simulink model "PropellerDynamics"  (R2024b)
settings: configuration reference "VTOLConfiguration" (kept outside this file)
undefined symbols (not defined in the file): minPWM, uavParam
libraries: sharedutil x2
settings Model: DataDictionary=VTOLDynamicsData.sldd  Creator=The MathWorks, Inc.  LastModifiedBy=jjha
settings ConfigSetRef: SourceName=VTOLConfiguration

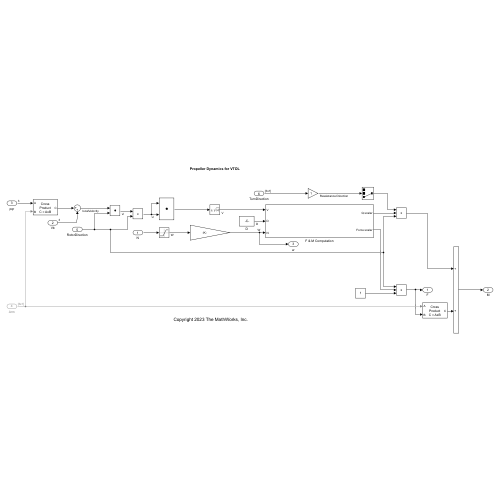
[thumbnail: Simulink's stored preview of the top-level diagram]
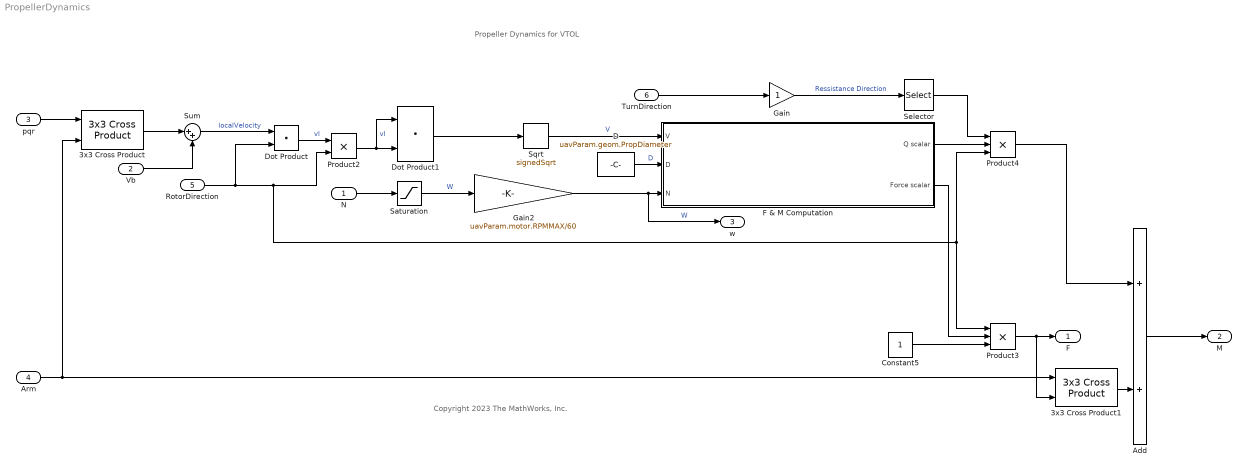
== system PropellerDynamics ==
  note: Propeller Dynamics for VTOL
  note: Copyright 2023 The MathWorks, Inc.
  N : Inport  OutDataTypeStr=double  PortDimensions=1
  Vb : Inport  Port=2  PortDimensions=3
  pqr : Inport  Port=3  PortDimensions=3
  Arm : Inport  Port=4  PortDimensions=[3 1]
  RotorDirection : Inport  Port=5
  TurnDirection : Inport  Port=6  PortDimensions=[3 1]
  3x3 Cross Product : sharedutil/3x3 Cross Product  aMode=aMode
  3x3 Cross Product1 : sharedutil/3x3 Cross Product  aMode=aMode
  Add : Sum
  Constant5 : Constant
  D : Constant  Value=uavParam.geom.PropDiameter
  Dot Product : DotProduct  OutDataTypeStr=Inherit: Inherit via internal rule
  Dot Product1 : DotProduct  OutDataTypeStr=Inherit: Inherit via internal rule
  F & M Computation : Subsystem
  Gain : Gain
  Gain2 : Gain  Gain=uavParam.motor.RPMMAX/60
  Product2 : Product
  Product3 : Product  Inputs=3
  Product4 : Product  Inputs=3
  Saturation : Saturate  UpperLimit=1  LowerLimit=minPWM
  Selector : Selector  InputPortWidth=3  IndexOptions=Index vector (dialog)  Indices=3  OutputSizes=1
  Sqrt : Sqrt  Operator=signedSqrt
  Sum : Sum  Inputs=|++
  F : Outport
  M : Outport  Port=2
  w : Outport  Port=3
  wires:
  3x3 Cross Product1/1 -> Add/2
  Sum/1 -> Dot Product/1  "localVelocity"
  N/1 -> Saturation/1
  pqr/1 -> 3x3 Cross Product/1
  Gain/1 -> Selector/1  "Ressistance Direction"
  Arm/1 -> 3x3 Cross Product/2, 3x3 Cross Product1/1
  Dot Product/1 -> Product2/1  "vl"
  3x3 Cross Product/1 -> Sum/1
  F & M Computation/2(Force scalar) -> Product3/2
  Vb/1 -> Sum/2
  RotorDirection/1 -> Product3/1, Product4/3, Product2/2, Dot Product/2
  Product2/1 -> Dot Product1/2, Dot Product1/1  "vl"
  Saturation/1 -> Gain2/1  "W"
  TurnDirection/1 -> Gain/1
  Dot Product1/1 -> Sqrt/1
  Sqrt/1 -> F & M Computation/1(V)  "V"
  D/1 -> F & M Computation/2(D)  "D"
  F & M Computation/1(Q scalar) -> Product4/2
  Selector/1 -> Product4/1
  Product3/1 -> 3x3 Cross Product1/2, F/1
  Constant5/1 -> Product3/3
  Product4/1 -> Add/1
  Add/1 -> M/1
  Gain2/1 -> w/1, F & M Computation/3(N)  "W"

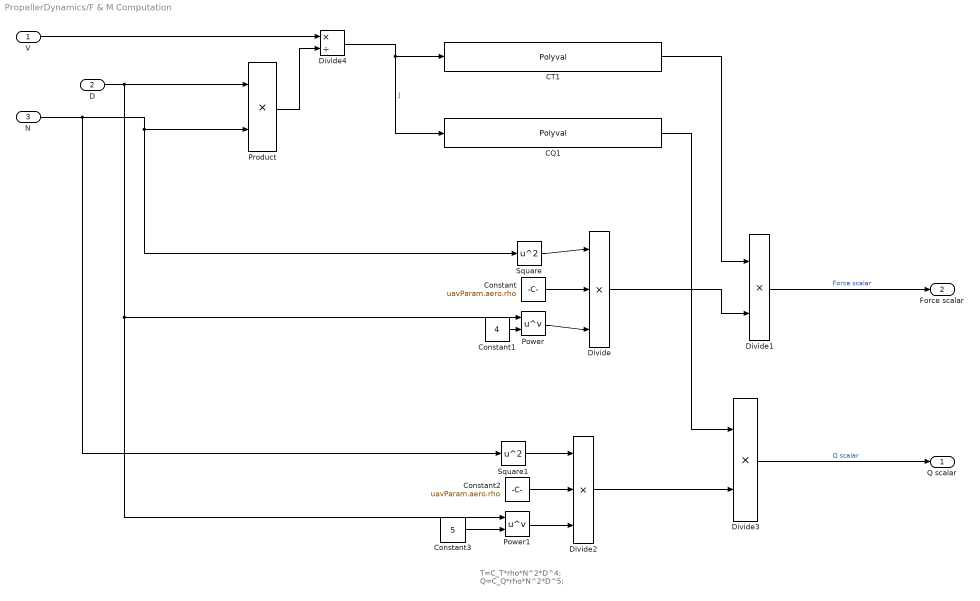
== system PropellerDynamics/F & M Computation ==
  note: T=C_T*rho*N^2*D^4;
      | Q=C_Q*rho*N^2*D^5;
  V : Inport
  D : Inport  Port=2
  N : Inport  Port=3
  CQ1 : Polyval  Coefs=[0.04280,-0.05046,0.005711,-0.003293, 0.007048]
  CT1 : Polyval  Coefs=[0.03338, -0.1265,-0.1210,0.1142]
  Constant : Constant  Value=uavParam.aero.rho
  Constant1 : Constant  Value=4
  Constant2 : Constant  Value=uavParam.aero.rho
  Constant3 : Constant  Value=5
  Divide : Product  Inputs=***
  Divide1 : Product  Inputs=**
  Divide2 : Product  Inputs=***
  Divide3 : Product  Inputs=**
  Divide4 : Product  Inputs=*/
  Power : Math  Operator=pow
  Power1 : Math  Operator=pow
  Product : Product
  Square : Math  Operator=square
  Square1 : Math  Operator=square
  Q scalar : Outport
  Force scalar : Outport  Port=2
  wires:
  Divide4/1 -> CQ1/1, CT1/1  "J"
  Product/1 -> Divide4/2
  CT1/1 -> Divide1/1
  Divide2/1 -> Divide3/2
  CQ1/1 -> Divide3/1
  Divide3/1 -> Q scalar/1  "Q scalar"
  Divide/1 -> Divide1/2
  Divide1/1 -> Force scalar/1  "Force scalar"
  V/1 -> Divide4/1
  Power/1 -> Divide/3
  Constant/1 -> Divide/2
  Constant3/1 -> Power1/2
  Square/1 -> Divide/1
  Power1/1 -> Divide2/3
  N/1 -> Square/1, Product/2, Square1/1
  D/1 -> Power/1, Power1/1, Product/1
  Constant1/1 -> Power/2
  Square1/1 -> Divide2/1
  Constant2/1 -> Divide2/2
